simulink model "Lab2_P3"  (R2019a)
settings: Solver=VariableStepAuto  StartTime=0.0  StopTime=10.0  RelTol=1e-3
settings Model: Creator=keeshigan  LastModifiedBy=keeshigan

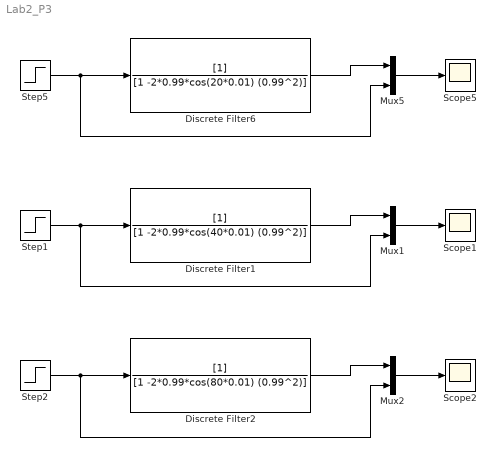
== system Lab2_P3 ==
  Discrete Filter1 : DiscreteFilter  Denominator=[1 -2*0.99*cos(40*0.01) (0.99^2)]  FilterStructure=Direct form I
  Discrete Filter2 : DiscreteFilter  Denominator=[1 -2*0.99*cos(80*0.01) (0.99^2)]  FilterStructure=Direct form I
  Discrete Filter6 : DiscreteFilter  Denominator=[1 -2*0.99*cos(20*0.01) (0.99^2)]  FilterStructure=Direct form I  SampleTime=0.01
  Mux1 : Mux  Inputs=2
  Mux2 : Mux  Inputs=2
  Mux5 : Mux  Inputs=2
  Scope1 : Scope
  Scope2 : Scope
  Scope5 : Scope
  Step1 : Step  SampleTime=0
  Step2 : Step  SampleTime=0
  Step5 : Step  SampleTime=0
  wires:
  Step5/1 -> Mux5/2, Discrete Filter6/1
  Discrete Filter6/1 -> Mux5/1
  Mux5/1 -> Scope5/1
  Step1/1 -> Mux1/2, Discrete Filter1/1
  Discrete Filter1/1 -> Mux1/1
  Mux1/1 -> Scope1/1
  Step2/1 -> Mux2/2, Discrete Filter2/1
  Discrete Filter2/1 -> Mux2/1
  Mux2/1 -> Scope2/1
